simulink model "PTC_MBDS_StringCompare_Sample"  (R2013a)
settings: Solver=FixedStepDiscrete  StartTime=0.0  StopTime=100  FixedStep=0.02  RelTol=1e-3
libraries: PTC_MBDS_LIB x2, simulink_extras x1
settings Model: BufferReuse=off  Creator=sundeep.tuteja  LastModifiedBy=sundeep.tuteja
settings OptimizationCC: BlockReduction=off  OptimizeBlockIOStorage=off  BufferReuse=off  ExpressionFolding=off  LocalBlockOutputs=off
settings HardwareCC: ProdIntDivRoundTo=Zero  ProdEndianess=LittleEndian  ProdHWDeviceType=Generic->Custom  TargetIntDivRoundTo=Zero  TargetEndianess=LittleEndian  TargetHWDeviceType=Generic->Custom
settings RTWCC: ProcessScript=grt_make_rtw_hook

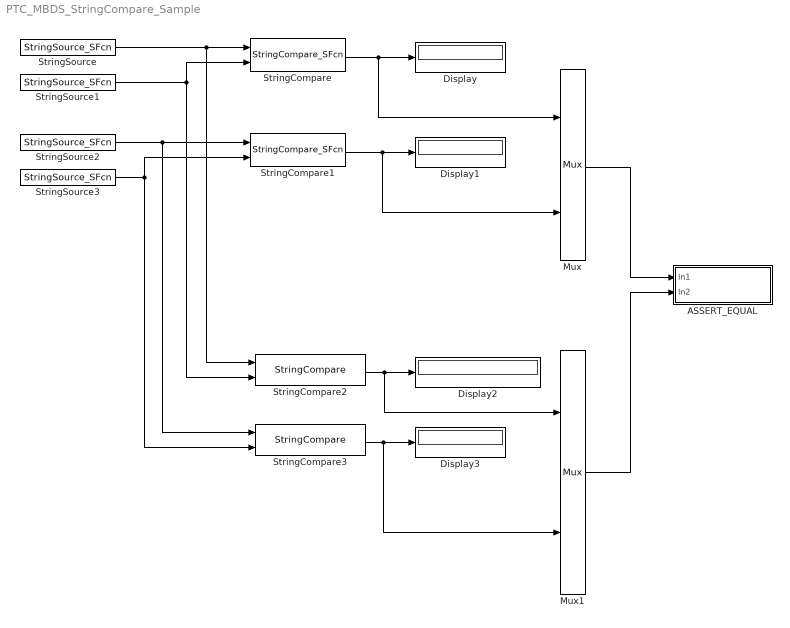
== system PTC_MBDS_StringCompare_Sample ==
  ASSERT_EQUAL : Subsystem
  Display{,1..3} (4 alike) : Display
  Mux : Mux  Inputs=2
  Mux1 : Mux  Inputs=2
  StringCompare : S-Function  InitFcn=|  FunctionName=StringCompare_SFcn  Parameters=uint16(MaxStringLength)  EnableBusSupport=off  mask(StringCompare){MBDS_LibraryBlock=on, MBDS_BlockVersion=05.40}
      | if(exist('MBDS_BlockCallback', 'file'))
      |    MBDS_BlockCallback('Update', gcb);
      | end
      mask prompts: MBDS_LibraryBlock "MBDS Library Block"; MBDS_BlockVersion "Block version:"
      mask help: The block compares two strings. If the two strings are equal the output is set to true, otherwise the output is set to false.
      mask init:
      | MBDS_BlockCallback('Copy', gcb);
      | MaxStringLength = 1 + GetStringLen();
      mask Help: eval(['open([workdir(''Library_Dir:''),''\Blockset\Help\'',get_param(gcb,''MaskType''),''.html''])'])
      mask Display:
      | disp('Compare')
      | port_label('input', 1, 'In1')
      | port_label('input', 2, 'In2')
      | port_label('output', 1, 'Out')
  StringCompare1 : S-Function  InitFcn=|  FunctionName=StringCompare_SFcn  Parameters=uint16(MaxStringLength)  EnableBusSupport=off  mask(StringCompare){MBDS_LibraryBlock=on, MBDS_BlockVersion=05.40}
      | if(exist('MBDS_BlockCallback', 'file'))
      |    MBDS_BlockCallback('Update', gcb);
      | end
      mask prompts: MBDS_LibraryBlock "MBDS Library Block"; MBDS_BlockVersion "Block version:"
      mask help: The block compares two strings. If the two strings are equal the output is set to true, otherwise the output is set to false.
      mask init:
      | MBDS_BlockCallback('Copy', gcb);
      | MaxStringLength = 1 + GetStringLen();
      mask Help: eval(['open([workdir(''Library_Dir:''),''\Blockset\Help\'',get_param(gcb,''MaskType''),''.html''])'])
      mask Display:
      | disp('Compare')
      | port_label('input', 1, 'In1')
      | port_label('input', 2, 'In2')
      | port_label('output', 1, 'Out')
  StringCompare2 : PTC_MBDS_LIB/MBDS Standard Library/Extended Operations/String Operations/StringCompare  PTC_MBDS_BlockVersion=5.32  PTC_BlockType=PTC_MBDS_StringCompare  MaxStringLength=PTC_MBDS_MaxStringLength_Fcn
  StringCompare3 : PTC_MBDS_LIB/MBDS Standard Library/Extended Operations/String Operations/StringCompare  PTC_MBDS_BlockVersion=5.32  PTC_BlockType=PTC_MBDS_StringCompare  MaxStringLength=PTC_MBDS_MaxStringLength_Fcn
  StringSource : S-Function  InitFcn=|  FunctionName=StringSource_SFcn  Parameters=uint8(String), uint16(MaxStringLength)  EnableBusSupport=off  mask(StringSource){MBDS_LibraryBlock=on, InputValue=MyString, MBDS_BlockVersion=05.31}
      | if(exist('MBDS_BlockCallback', 'file'))
      |    MBDS_BlockCallback('Update', gcb);
      | end
      mask prompts: MBDS_LibraryBlock "MBDS Library Block"; InputValue "Constant value:"; MBDS_BlockVersion "Block version:"
      mask help: This block outputs an uint8 array based on the ASCII codes of the string specified by the user.
      mask init:
      | MBDS_BlockCallback('Copy', gcb);
      | MaxStringLength = 1 + GetStringLen();
      | DispString = 'Error';
      | String = InputValue;
      | % Skip if string specifies a numeric expression or starts with '
      | if(isempty(str2num(String)) && String(1) ~= '''')
      |    try
      |       % Try to evaluate project constant 
      |       String = evalin('base', String);
      |    end   
      | end
      | if ~ischar(String) || size(String, 1) > 1
      | 	error('String must be a [1xn] array of type ''char'' with at least one character')
      | else
      |    % Limit to max. string length
      |    String = String(1:min(MaxStringLength, length(String)));
      | 	DispString = InputValue;
      | end
      mask Help: eval(['open([workdir(''Library_Dir:''),''\Blockset\Help\'',get_param(gcb,''MaskType''),''.html''])'])
      mask Display: text(0.05,0.5,DispString,'horizontalAlignment','left')
  StringSource1 : S-Function  InitFcn=|  FunctionName=StringSource_SFcn  Parameters=uint8(String), uint16(MaxStringLength)  EnableBusSupport=off  mask(StringSource){MBDS_LibraryBlock=on, InputValue=MyString, MBDS_BlockVersion=05.31}
      | if(exist('MBDS_BlockCallback', 'file'))
      |    MBDS_BlockCallback('Update', gcb);
      | end
      mask prompts: MBDS_LibraryBlock "MBDS Library Block"; InputValue "Constant value:"; MBDS_BlockVersion "Block version:"
      mask help: This block outputs an uint8 array based on the ASCII codes of the string specified by the user.
      mask init: same as PTC_MBDS_StringCompare_Sample/StringSource
      mask Help: eval(['open([workdir(''Library_Dir:''),''\Blockset\Help\'',get_param(gcb,''MaskType''),''.html''])'])
      mask Display: text(0.05,0.5,DispString,'horizontalAlignment','left')
  StringSource2 : S-Function  InitFcn=|  FunctionName=StringSource_SFcn  Parameters=uint8(String), uint16(MaxStringLength)  EnableBusSupport=off  mask(StringSource){MBDS_LibraryBlock=on, InputValue=MyString, MBDS_BlockVersion=05.31}
      | if(exist('MBDS_BlockCallback', 'file'))
      |    MBDS_BlockCallback('Update', gcb);
      | end
      mask prompts: MBDS_LibraryBlock "MBDS Library Block"; InputValue "Constant value:"; MBDS_BlockVersion "Block version:"
      mask help: This block outputs an uint8 array based on the ASCII codes of the string specified by the user.
      mask init: same as PTC_MBDS_StringCompare_Sample/StringSource
      mask Help: eval(['open([workdir(''Library_Dir:''),''\Blockset\Help\'',get_param(gcb,''MaskType''),''.html''])'])
      mask Display: text(0.05,0.5,DispString,'horizontalAlignment','left')
  StringSource3 : S-Function  InitFcn=|  FunctionName=StringSource_SFcn  Parameters=uint8(String), uint16(MaxStringLength)  EnableBusSupport=off  mask(StringSource){MBDS_LibraryBlock=on, InputValue=MyString, MBDS_BlockVersion=05.31}
      | if(exist('MBDS_BlockCallback', 'file'))
      |    MBDS_BlockCallback('Update', gcb);
      | end
      mask prompts: MBDS_LibraryBlock "MBDS Library Block"; InputValue "Constant value:"; MBDS_BlockVersion "Block version:"
      mask help: This block outputs an uint8 array based on the ASCII codes of the string specified by the user.
      mask init: same as PTC_MBDS_StringCompare_Sample/StringSource
      mask Help: eval(['open([workdir(''Library_Dir:''),''\Blockset\Help\'',get_param(gcb,''MaskType''),''.html''])'])
      mask Display: text(0.05,0.5,DispString,'horizontalAlignment','left')
  wires:
  StringSource/1 -> StringCompare/1, StringCompare2/1
  StringSource1/1 -> StringCompare/2, StringCompare2/2
  StringSource2/1 -> StringCompare1/1, StringCompare3/1
  StringSource3/1 -> StringCompare1/2, StringCompare3/2
  Mux/1 -> ASSERT_EQUAL/1(In1)
  Mux1/1 -> ASSERT_EQUAL/2(In2)
  StringCompare/1 -> Mux/1, Display/1
  StringCompare1/1 -> Mux/2, Display1/1
  StringCompare2/1 -> Mux1/1, Display2/1
  StringCompare3/1 -> Mux1/2, Display3/1

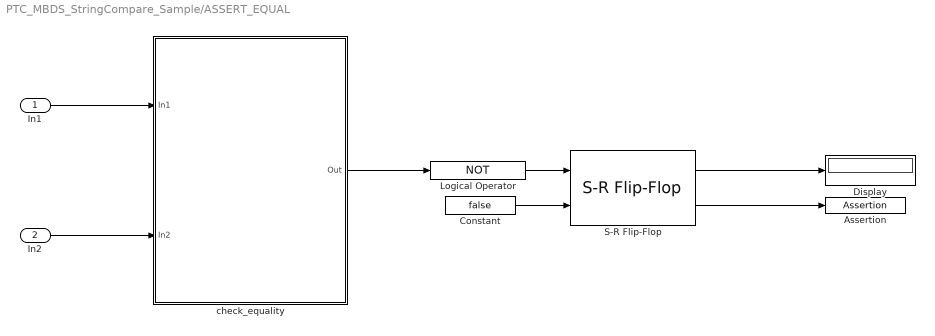
== system PTC_MBDS_StringCompare_Sample/ASSERT_EQUAL ==
  In1 : Inport
  In2 : Inport  Port=2
  Assertion : Assertion
  Constant : Constant  Value=false
  Display : Display
  Logical Operator : Logic  Operator=NOT  AllPortsSameDT=off  OutDataTypeStr=boolean
  S-R Flip-Flop : simulink_extras/Flip Flops/S-R Flip-Flop  initial_condition=0
  check_equality : MATLAB Function  TreatAsAtomicUnit=on
  wires:
  S-R Flip-Flop/1 -> Display/1
  check_equality/1(Out) -> Logical Operator/1
  Constant/1 -> S-R Flip-Flop/2
  S-R Flip-Flop/2 -> Assertion/1
  In2/1 -> check_equality/2(In2)
  In1/1 -> check_equality/1(In1)
  Logical Operator/1 -> S-R Flip-Flop/1

== matlab function PTC_MBDS_StringCompare_Sample/ASSERT_EQUAL/check_equality ==
  data: In1 input; Out output; In2 input
function Out = check_equality(In1, In2)
%#codegen

Out = isequaln(In1, In2);

end
